simulink model "test_pi_av_formation_gazebo_final_variation"  (R2023a)
settings: Solver=FixedStepAuto  StartTime=0.0  StopTime=inf  FixedStep=0.07  RelTol=1e-3
undefined symbols (not defined in the file or in its folder): angular, DiscIntNeverNeededParam, linear
libraries: ros2lib x14, simulink x4, robotcorelib x4
(part 2 of 2)

== matlab function test_pi_av_formation_gazebo_final_variation/Translational Control2/Flocking1/MATLAB Function2 ==
  data: ui_prev input; xi input; yi input; zi input; ui_gamma output; xr input; yr input; zr input; xr2 input; yr2 input; zr2 input; fig input; iep input size=3; norm_ex input; norm_ey input; norm_ez input; ep output size=3; K_cts input

function [ui_gamma, ep] = naviFeedback(ui_prev, xi, yi, zi, xr, yr, zr, xr2, yr2, zr2, fig, iep, norm_ex, norm_ey, norm_ez, K_cts)
    
    Kpxy = K_cts(1); Kixy = K_cts(2);
    xmin_xy = K_cts(3); xmax_xy = K_cts(4);
    Kpz = K_cts(5); Kiz = K_cts(6);
    xmin_z = K_cts(7); xmax_z = K_cts(8);

    %Sepration control
    ui_xprev = ui_prev(1); ui_yprev = ui_prev(2); ui_zprev = ui_prev(3);
    
    if fig == 1
        e_x = (xr - xi - 0.5) + (xr2 - xi - 1);
        e_y = (yr - yi + 0.5) + (yr2 - yi + 1);
        e_z = (zr - zi - 0.1) + (zr2 - zi);
    elseif fig == 2
        e_x = (xr - xi - 0.5) + (xr2 - xi - 1);
        e_y = (yr - yi - 0.5) + (yr2 - yi - 1);
        e_z = (zr - zi + 0.1) + (zr2 - zi);
    else
        e_x = (xr - xi - 0.5) + (xr2 - xi - 1);
        e_y = (yr - yi - 0.5) + (yr2 - yi - 1);
        e_z = (zr - zi + 0.1) + (zr2 - zi);
    end

    e_xy = [e_x;e_y];
    ep = [e_xy;e_z];
    
    if  norm_ex >= 0
        ui_gammax = satFcn_esc(Kpxy*e_x, xmin_xy, xmax_xy) + satFcn_esc(Kixy*iep(1), xmin_xy, xmax_xy);
    else
        ui_gammax = ui_xprev;
    end

    if  norm_ey >= 0
        ui_gammay = satFcn_esc(Kpxy*e_y, xmin_xy, xmax_xy) + satFcn_esc(Kixy*iep(1), xmin_xy, xmax_xy);
    else
        ui_gammay = ui_yprev;
    end

    if  norm_ez >= 0
        ui_gammaz = satFcn_esc(Kpz*e_z, xmin_z, xmax_z) + satFcn_esc(Kiz*iep(3), xmin_z, xmax_z);
    else
        ui_gammaz = ui_zprev;
    end
    

    ui_gamma = [ui_gammax;ui_gammay;ui_gammaz];
    
end

== matlab function test_pi_av_formation_gazebo_final_variation/Translational Control3/Flocking1/MATLAB Function ==
  data: xi input; yi input; phiAlpha output; xj input; yj input; xk input; yk input; xl input; yl input; params input

function phiAlpha  = phiAlphaFcn(xi, yi, xj, yj, xk, yk, xl, yl, params)
    
    % Flocking parameters
    epsilon = params(1); a = params(2); b = params(3); c = params(4); d = params(5); h = params(6);

    e = abs(a - b) / sqrt(4*a*b) ;

    cAlpha = sigmaNormFun(c, epsilon) ;
    dAlpha = sigmaNormFun(d, epsilon) ;

    %%
    Pi = [xi;yi] ;
    Pj = [xj;yj] ;
    Pk = [xk;yk] ;
    Pl = [xl;yl] ;

    %%
    sigmaNormj = sigmaNormFun(Pj - Pi, epsilon) ;
    nij = gradSigmaFun(Pj - Pi, epsilon) ;
    
    sigmaNormk = sigmaNormFun(Pk - Pi, epsilon) ;
    nik = gradSigmaFun(Pk - Pi, epsilon) ;

    sigmaNorml = sigmaNormFun(Pl - Pi, epsilon) ;
    nil = gradSigmaFun(Pl - Pi, epsilon) ;

    %%
    sigma1j = sigma1Fun(sigmaNormj - dAlpha + e) ;
    sigma1k = sigma1Fun(sigmaNormk - dAlpha + e) ;
    sigma1l = sigma1Fun(sigmaNorml - dAlpha + e) ;
            
    %% Position
    phiAlphaj = 0.5 * bumpFcn(sigmaNormj/cAlpha,h) * ((a+b)*sigma1j + (a-b)) ;
    phiAlphanij = phiAlphaj.* nij ;
    
    phiAlphak = 0.5 * bumpFcn(sigmaNormk/cAlpha,h) * ((a+b)*sigma1k + (a-b)) ;
    phiAlphanik = phiAlphak.* nik ;

    phiAlphal = 0.5 * bumpFcn(sigmaNorml/cAlpha,h) * ((a+b)*sigma1l + (a-b)) ;
    phiAlphanil = phiAlphal.* nil ;

    phiAlpha = phiAlphanij + phiAlphanik + phiAlphanil;

    
end

== matlab function test_pi_av_formation_gazebo_final_variation/Translational Control3/Flocking1/MATLAB Function1 ==
  data: eta input; phiAlpha input; phiAlpha_int input; ui_gamma input; yaw input; Ui_pos output size=3; ui_yaw output; KP input; eyaw output size=1; eyaw1 input; eyaw2 input; eyaw4 input

function [Ui_pos, ui_yaw, eyaw]  = ctrlLaw(eta, phiAlpha, phiAlpha_int, ui_gamma, yaw, KP, eyaw1, eyaw2, eyaw4)  %, phiBetak, bikobs, phiBetanei, bikve
    
    % Control gains and parameters
    Kx = KP(1); Ky = KP(2); Kz = KP(3);
    Kix = KP(4); Kiy = KP(5); Kiz = KP(6);
    Kyaw = KP(7); Kdyaw = KP(8);
    off = KP(9);

    eyaw = 0 - yaw(1);
    deyaw = 0 - yaw(2);


    ui_yaw = Kyaw*eyaw + Kdyaw*deyaw;
    hz_dot = ui_gamma(3,1) - eta(3,1);  %+ cBetaz * (phiBetak(3,1) + phiBetanei(3,1)) + cdBetaz * (bikobs(3,1) + bikve(3,1));

    if eyaw < off && eyaw > -off % && eyaw1 < off && eyaw1 > -off && eyaw2 < off && eyaw2 > -off && eyaw4 < off && eyaw4 > -off
        hx_dot = Kx * phiAlpha(1,1) + Kix * phiAlpha_int(1,1) + ui_gamma(1,1) - eta(1,1);  %+ cBetax * (phiBetak(1,1) + phiBetanei(1,1)) + cdBetax * (bikobs(1,1) + bikve(1,1));
        hy_dot = Ky * phiAlpha(2,1) + Kiy * phiAlpha_int(2,1) + ui_gamma(2,1) - eta(2,1);  %+ cBetay * (phiBetak(2,1) + phiBetanei(2,1)) + cdBetay * (bikobs(2,1) + bikve(2,1));
    else
        hx_dot = 0;
        hy_dot = 0;
    end
    

    Ui_pos = [hx_dot; hy_dot; hz_dot] ;
    

end

== matlab function test_pi_av_formation_gazebo_final_variation/Translational Control3/Flocking1/MATLAB Function2 ==
  data: ui_prev input; xi input; yi input; zi input; ui_gamma output; xr input; yr input; zr input; xr2 input; yr2 input; zr2 input; fig input; iep input size=3; norm_ex input; norm_ey input; norm_ez input; ep output size=3; K_cts input
function [ui_gamma, ep] = naviFeedback(ui_prev, xi, yi, zi, xr, yr, zr, xr2, yr2, zr2, fig, iep, norm_ex, norm_ey, norm_ez, K_cts)
    
    Kpxy = K_cts(1); Kixy = K_cts(2);
    xmin_xy = K_cts(3); xmax_xy = K_cts(4);
    Kpz = K_cts(5); Kiz = K_cts(6);
    xmin_z = K_cts(7); xmax_z = K_cts(8);

    %Sepration control
    ui_xprev = ui_prev(1); ui_yprev = ui_prev(2); ui_zprev = ui_prev(3);

    
    if fig == 1
        e_x = (xr - xi - 0.5) + (xr2 - xi - 1);
        e_y = (yr - yi - 0.5) + (yr2 - yi);
        e_z = (zr - zi + 0.1) + (zr2 - zi);
    elseif fig == 2
        e_x = (xr - xi + 0.5) + (xr2 - xi);
        e_y = (yr - yi - 0.5) + (yr2 - yi - 1);
        e_z = (zr - zi - 0.1) + (zr2 - zi);
    else
        e_x = (xr - xi + 0.5) + (xr2 - xi);
        e_y = (yr - yi - 0.5) + (yr2 - yi - 1);
        e_z = (zr - zi - 0.5) + (zr2 - zi - 0.6);
    end

    e_xy = [e_x;e_y];
    ep = [e_xy;e_z];
    
    if  norm_ex >= 0
        ui_gammax = satFcn_esc(Kpxy*e_x, xmin_xy, xmax_xy) + satFcn_esc(Kixy*iep(1), xmin_xy, xmax_xy);
    else
        ui_gammax = ui_xprev;
    end

    if  norm_ey >= 0
        ui_gammay = satFcn_esc(Kpxy*e_y, xmin_xy, xmax_xy) + satFcn_esc(Kixy*iep(1), xmin_xy, xmax_xy);
    else
        ui_gammay = ui_yprev;
    end

    if  norm_ez >= 0
        ui_gammaz = satFcn_esc(Kpz*e_z, xmin_z, xmax_z) + satFcn_esc(Kiz*iep(3), xmin_z, xmax_z);
    else
        ui_gammaz = ui_zprev;
    end
    

    ui_gamma = [ui_gammax;ui_gammay;ui_gammaz];
end

== matlab function test_pi_av_formation_gazebo_final_variation/Translational Control4/Flocking1/MATLAB Function ==
  data: xi input; yi input; phiAlpha output; xj input; yj input; xk input; yk input; xl input; yl input; params input

function phiAlpha  = phiAlphaFcn(xi, yi, xj, yj, xk, yk, xl, yl, params)
    
    % Flocking parameters
    epsilon = params(1); a = params(2); b = params(3); c = params(4); d = params(5); h = params(6);

    e = abs(a - b) / sqrt(4*a*b) ;

    cAlpha = sigmaNormFun(c, epsilon) ;
    dAlpha = sigmaNormFun(d, epsilon) ;

    %%
    Pi = [xi;yi] ;
    Pj = [xj;yj] ;
    Pk = [xk;yk] ;
    Pl = [xl;yl] ;

    %%
    sigmaNormj = sigmaNormFun(Pj - Pi, epsilon) ;
    nij = gradSigmaFun(Pj - Pi, epsilon) ;
    
    sigmaNormk = sigmaNormFun(Pk - Pi, epsilon) ;
    nik = gradSigmaFun(Pk - Pi, epsilon) ;

    sigmaNorml = sigmaNormFun(Pl - Pi, epsilon) ;
    nil = gradSigmaFun(Pl - Pi, epsilon) ;

    %%
    sigma1j = sigma1Fun(sigmaNormj - dAlpha + e) ;
    sigma1k = sigma1Fun(sigmaNormk - dAlpha + e) ;
    sigma1l = sigma1Fun(sigmaNorml - dAlpha + e) ;
            
    %% Position
    phiAlphaj = 0.5 * bumpFcn(sigmaNormj/cAlpha,h) * ((a+b)*sigma1j + (a-b)) ;
    phiAlphanij = phiAlphaj.* nij ;
    
    phiAlphak = 0.5 * bumpFcn(sigmaNormk/cAlpha,h) * ((a+b)*sigma1k + (a-b)) ;
    phiAlphanik = phiAlphak.* nik ;

    phiAlphal = 0.5 * bumpFcn(sigmaNorml/cAlpha,h) * ((a+b)*sigma1l + (a-b)) ;
    phiAlphanil = phiAlphal.* nil ;

    phiAlpha = phiAlphanij + phiAlphanik + phiAlphanil;

    
end

== matlab function test_pi_av_formation_gazebo_final_variation/Translational Control4/Flocking1/MATLAB Function1 ==
  data: eta input; phiAlpha input; phiAlpha_int input; ui_gamma input; yaw input; Ui_pos output size=3; ui_yaw output; KP input; eyaw output size=1; eyaw1 input; eyaw2 input; eyaw3 input

function [Ui_pos, ui_yaw, eyaw]  = ctrlLaw(eta, phiAlpha, phiAlpha_int, ui_gamma, yaw, KP, eyaw1, eyaw2, eyaw3)  %, phiBetak, bikobs, phiBetanei, bikve
    
    % Control gains and parameters
    Kx = KP(1); Ky = KP(2); Kz = KP(3);
    Kix = KP(4); Kiy = KP(5); Kiz = KP(6);
    Kyaw = KP(7); Kdyaw = KP(8);
    off = KP(9);

    eyaw = 0 - yaw(1);
    deyaw = 0 - yaw(2);


    ui_yaw = Kyaw*eyaw + Kdyaw*deyaw;
    hz_dot = ui_gamma(3,1) - eta(3,1);  %+ cBetaz * (phiBetak(3,1) + phiBetanei(3,1)) + cdBetaz * (bikobs(3,1) + bikve(3,1));

    if eyaw < off && eyaw > -off % && eyaw1 < off && eyaw1 > -off && eyaw2 < off && eyaw2 > -off && eyaw3 < off && eyaw3 > -off
        hx_dot = Kx * phiAlpha(1,1) + Kix * phiAlpha_int(1,1) + ui_gamma(1,1) - eta(1,1);  %+ cBetax * (phiBetak(1,1) + phiBetanei(1,1)) + cdBetax * (bikobs(1,1) + bikve(1,1));
        hy_dot = Ky * phiAlpha(2,1) + Kiy * phiAlpha_int(2,1) + ui_gamma(2,1) - eta(2,1);  %+ cBetay * (phiBetak(2,1) + phiBetanei(2,1)) + cdBetay * (bikobs(2,1) + bikve(2,1));
    else
        hx_dot = 0;
        hy_dot = 0;
    end
    

    Ui_pos = [hx_dot; hy_dot; hz_dot] ;
    

end

== matlab function test_pi_av_formation_gazebo_final_variation/Translational Control1/Flocking1/MATLAB Function ==
  data: xi input; yi input; phiAlpha output; xj input; yj input; xk input; yk input; xl input; yl input; params input

function phiAlpha  = phiAlphaFcn(xi, yi, xj, yj, xk, yk, xl, yl, params)
    
    % Flocking parameters
    epsilon = params(1); a = params(2); b = params(3); c = params(4); d = params(5); h = params(6);

    e = abs(a - b) / sqrt(4*a*b) ;

    cAlpha = sigmaNormFun(c, epsilon) ;
    dAlpha = sigmaNormFun(d, epsilon) ;

    %%
    Pi = [xi;yi] ;
    Pj = [xj;yj] ;
    Pk = [xk;yk] ;
    Pl = [xl;yl] ;

    %%
    sigmaNormj = sigmaNormFun(Pj - Pi, epsilon) ;
    nij = gradSigmaFun(Pj - Pi, epsilon) ;
    
    sigmaNormk = sigmaNormFun(Pk - Pi, epsilon) ;
    nik = gradSigmaFun(Pk - Pi, epsilon) ;

    sigmaNorml = sigmaNormFun(Pl - Pi, epsilon) ;
    nil = gradSigmaFun(Pl - Pi, epsilon) ;

    %%
    sigma1j = sigma1Fun(sigmaNormj - dAlpha + e) ;
    sigma1k = sigma1Fun(sigmaNormk - dAlpha + e) ;
    sigma1l = sigma1Fun(sigmaNorml - dAlpha + e) ;
            
    %% Position
    phiAlphaj = 0.5 * bumpFcn(sigmaNormj/cAlpha,h) * ((a+b)*sigma1j + (a-b)) ;
    phiAlphanij = phiAlphaj.* nij ;
    
    phiAlphak = 0.5 * bumpFcn(sigmaNormk/cAlpha,h) * ((a+b)*sigma1k + (a-b)) ;
    phiAlphanik = phiAlphak.* nik ;

    phiAlphal = 0.5 * bumpFcn(sigmaNorml/cAlpha,h) * ((a+b)*sigma1l + (a-b)) ;
    phiAlphanil = phiAlphal.* nil ;

    phiAlpha = phiAlphanij + phiAlphanik + phiAlphanil;

    
end

== matlab function test_pi_av_formation_gazebo_final_variation/Translational Control1/Flocking1/MATLAB Function1 ==
  data: eta input; phiAlpha input; phiAlpha_int input; ui_gamma input; yaw input; Ui_pos output size=3; ui_yaw output; KP input; eyaw output size=1; eyaw2 input; eyaw3 input; eyaw4 input

function [Ui_pos, ui_yaw, eyaw]  = ctrlLaw(eta, phiAlpha, phiAlpha_int, ui_gamma, yaw, KP, eyaw2, eyaw3, eyaw4)  %, phiBetak, bikobs, phiBetanei, bikve
    
    % Control gains and parameters
    Kx = KP(1); Ky = KP(2); Kz = KP(3);
    Kix = KP(4); Kiy = KP(5); Kiz = KP(6);
    Kyaw = KP(7); Kdyaw = KP(8);
    off = KP(9);


    eyaw = 0 - yaw(1);
    deyaw = 0 - yaw(2);


    ui_yaw = Kyaw*eyaw + Kdyaw*deyaw;
    hz_dot = ui_gamma(3,1) - eta(3,1);  %+ cBetaz * (phiBetak(3,1) + phiBetanei(3,1)) + cdBetaz * (bikobs(3,1) + bikve(3,1));

    if eyaw < off && eyaw > -off % && eyaw2 < off && eyaw2 > -off  && eyaw3 < off && eyaw3 > -off && eyaw4 < off && eyaw4 > -off
        hx_dot = Kx * phiAlpha(1,1) + Kix * phiAlpha_int(1,1) + ui_gamma(1,1) - eta(1,1);  %+ cBetax * (phiBetak(1,1) + phiBetanei(1,1)) + cdBetax * (bikobs(1,1) + bikve(1,1));
        hy_dot = Ky * phiAlpha(2,1) + Kiy * phiAlpha_int(2,1) + ui_gamma(2,1) - eta(2,1);  %+ cBetay * (phiBetak(2,1) + phiBetanei(2,1)) + cdBetay * (bikobs(2,1) + bikve(2,1));
    else
        hx_dot = 0;
        hy_dot = 0;
    end
    

    Ui_pos = [hx_dot; hy_dot; hz_dot] ;
    

end

== matlab function test_pi_av_formation_gazebo_final_variation/Translational Control1/Flocking1/MATLAB Function2 ==
  data: ui_prev input; xi input; yi input; zi input; ui_gamma output; xr input; yr input; zr input; figure input; iep input size=3; norm_ex input; norm_ey input; norm_ez input; ep output size=3; K_cts input

function [ui_gamma, ep] = naviFeedback(ui_prev, xi, yi, zi, xr, yr, zr, figure, iep, norm_ex, norm_ey, norm_ez, K_cts)
    
    Kpxy = K_cts(1); Kixy = K_cts(2);
    xmin_xy = K_cts(3); xmax_xy = K_cts(4);
    Kpz = K_cts(5); Kiz = K_cts(6);
    xmin_z = K_cts(7); xmax_z = K_cts(8);

    %Sepration control
    ui_xprev = ui_prev(1); ui_yprev = ui_prev(2); ui_zprev = ui_prev(3);

    if figure == 1
        e_x = xr - xi + 0.5;
        e_y = yr - yi + 0.5;
        e_z = zr - zi + 0.1;
    elseif figure == 2
        e_x = xr - xi - 0.5;
        e_y = yr - yi + 0.5;
        e_z = zr - zi - 0.1;
    else
        e_x = xr - xi - 0.5;
        e_y = yr - yi + 0.5;
        e_z = zr - zi - 0.5;
    end

    e_xy = [e_x;e_y];
    ep = [e_xy;e_z];
    
    if  norm_ex >= 0
        ui_gammax = satFcn_esc(Kpxy*e_x, xmin_xy, xmax_xy) + satFcn_esc(Kixy*iep(1), xmin_xy, xmax_xy);
    else
        ui_gammax = ui_xprev;
    end

    if  norm_ey >= 0
        ui_gammay = satFcn_esc(Kpxy*e_y, xmin_xy, xmax_xy) + satFcn_esc(Kixy*iep(1), xmin_xy, xmax_xy);
    else
        ui_gammay = ui_yprev;
    end

    if  norm_ez >= 0
        ui_gammaz = satFcn_esc(Kpz*e_z, xmin_z, xmax_z) + satFcn_esc(Kiz*iep(3), xmin_z, xmax_z);
    else
        ui_gammaz = ui_zprev;
    end
    

    ui_gamma = [ui_gammax;ui_gammay;ui_gammaz];
    
end

== matlab function test_pi_av_formation_gazebo_final_variation/Translational Control4/Flocking1/MATLAB Function2 ==
  data: ui_prev input; xi input; yi input; zi input; ui_gamma output; xr input; yr input; zr input; xr2 input; yr2 input; zr2 input; fig input; iep input size=3; norm_ex input; norm_ey input; norm_ez input; ep output size=3; K_cts input
function [ui_gamma, ep] = naviFeedback(ui_prev, xi, yi, zi, xr, yr, zr, xr2, yr2, zr2, fig, iep, norm_ex, norm_ey, norm_ez, K_cts)
    
    Kpxy = K_cts(1); Kixy = K_cts(2);
    xmin_xy = K_cts(3); xmax_xy = K_cts(4);
    Kpz = K_cts(5); Kiz = K_cts(6);
    xmin_z = K_cts(7); xmax_z = K_cts(8);

    %Sepration control
    ui_xprev = ui_prev(1); ui_yprev = ui_prev(2); ui_zprev = ui_prev(3);
    
    if fig == 1
        e_x = (xr - xi + 0.5) + (xr2 - xi);
        e_y = (yr - yi - 0.5) + (yr2 - yi - 1);
        e_z = (zr - zi - 0.1) + (zr2 - zi);
    elseif fig == 2
        e_x = (xr - xi + 0.5) + (xr2 - xi + 1);
        e_y = (yr - yi + 0.5) + (yr2 - yi);
        e_z = (zr - zi + 0.1) + (zr2 - zi);
    else
        e_x = (xr - xi + 0.5) + (xr2 - xi + 1);
        e_y = (yr - yi + 0.5) + (yr2 - yi);
        e_z = (zr - zi + 0.1) + (zr2 - zi);
    end

    e_xy = [e_x;e_y];
    ep = [e_xy;e_z];
    
    if  norm_ex >= 0
        ui_gammax = satFcn_esc(Kpxy*e_x, xmin_xy, xmax_xy) + satFcn_esc(Kixy*iep(1), xmin_xy, xmax_xy);
    else
        ui_gammax = ui_xprev;
    end

    if  norm_ey >= 0
        ui_gammay = satFcn_esc(Kpxy*e_y, xmin_xy, xmax_xy) + satFcn_esc(Kixy*iep(1), xmin_xy, xmax_xy);
    else
        ui_gammay = ui_yprev;
    end

    if  norm_ez >= 0
        ui_gammaz = satFcn_esc(Kpz*e_z, xmin_z, xmax_z) + satFcn_esc(Kiz*iep(3), xmin_z, xmax_z);
    else
        ui_gammaz = ui_zprev;
    end
    

    ui_gamma = [ui_gammax;ui_gammay;ui_gammaz];
end

== matlab function test_pi_av_formation_gazebo_final_variation/Translational Control1/Flocking1/MATLAB Function5 ==
  data: dot_hat_q output; L input; q input; q_hat input; eta1 input; u input; dot_eta output
function [dot_hat_q, dot_eta] = fcn(L, q, q_hat, eta1, u)

%%separation gains vectors
l1 = [L(1) L(2) L(3)];
l0 = [L(4) L(5) L(6)];

L_1 = diag(l1);
L_0 = diag(l0);

dot_hat_q = q_est(u, eta1, L_1, q, q_hat);

dot_eta = dot_eta_two(L_0, q, q_hat);

== matlab function test_pi_av_formation_gazebo_final_variation/Translational Control2/Flocking1/MATLAB Function5 ==
  data: dot_hat_q output; L input; q input; q_hat input; eta1 input; u input; dot_eta output
function [dot_hat_q, dot_eta] = fcn(L, q, q_hat, eta1, u)

%%separation gains vectors
l1 = [L(1) L(2) L(3)];
l0 = [L(4) L(5) L(6)];

L_1 = diag(l1);
L_0 = diag(l0);

dot_hat_q = q_est(u, eta1, L_1, q, q_hat);

dot_eta = dot_eta_two(L_0, q, q_hat);

== matlab function test_pi_av_formation_gazebo_final_variation/Translational Control3/Flocking1/MATLAB Function5 ==
  data: dot_hat_q output; L input; q input; q_hat input; eta1 input; u input; dot_eta output
function [dot_hat_q, dot_eta] = fcn(L, q, q_hat, eta1, u)

%%separation gains vectors
l1 = [L(1) L(2) L(3)];
l0 = [L(4) L(5) L(6)];

L_1 = diag(l1);
L_0 = diag(l0);

dot_hat_q = q_est(u, eta1, L_1, q, q_hat);

dot_eta = dot_eta_two(L_0, q, q_hat);

== matlab function test_pi_av_formation_gazebo_final_variation/Translational Control4/Flocking1/MATLAB Function5 ==
  data: dot_hat_q output; L input; q input; q_hat input; eta1 input; u input; dot_eta output
function [dot_hat_q, dot_eta] = fcn(L, q, q_hat, eta1, u)

%%separation gains vectors
l1 = [L(1) L(2) L(3)];
l0 = [L(4) L(5) L(6)];

L_1 = diag(l1);
L_0 = diag(l0);

dot_hat_q = q_est(u, eta1, L_1, q, q_hat);

dot_eta = dot_eta_two(L_0, q, q_hat);

== matlab function test_pi_av_formation_gazebo_final_variation/Translational Control1/Flocking1/event_x2 ==
  data: e_1 output; e_2 output; e1 input; e2 input; e3 input; e_3 output; i1 output; i1 input; i2 input; i3 input; i2 output; i3 output
function [e_1,e_2, e_3, i1, i2, i3]  = fcn(e1, e2, e3, i1, i2, i3)

if e1 >= 0
    e_1 = 1;
    i1 = i1+1;
else 
    e_1 = 0;
    i1 = i1;
end

if e2 >= 0
    e_2 = 1;
    i2 = i2 + 1;
else 
    e_2 = 0;
    i2 = i2;
end

if e3 >= 0
    e_3 = 1;
    i3 = i3 + 1;
else 
    e_3 = 0;
    i3 = i3;
end

== matlab function test_pi_av_formation_gazebo_final_variation/Translational Control1/Flocking1/event_1 ==
  data: x input; y input; z input; mx input; my input; mz input; norm_ex output; norm_ey output; c0 input; norm_ez output
function [norm_ex, norm_ey, norm_ez] = fcn(x, y, z, mx, my, mz, c0)

cx = c0(1); cy = c0(2); cz = c0(3); 

norm_ex = abs((mx-x)) - cx;
norm_ey = abs((my-y)) - cy;
norm_ez = abs((mz-z)) - cz;

== matlab function test_pi_av_formation_gazebo_final_variation/Translational Control1/Flocking1/memory_1 ==
  data: ex input; ey input; mx output; ez input; x input; y input; z input; mx input; my input; mz input; my output; mz output
function [mx, my, mz] = fcn(ex, ey, ez, x, y, z, mx, my, mz)

if ex >= 0
    mx = x;    
else
    mx = mx;
end

if ey >= 0
    my = y;    
else
    my = my;
end

if ez >= 0
    mz = z;    
else
    mz = mz;
end

== matlab function test_pi_av_formation_gazebo_final_variation/Translational Control2/Flocking1/event_1 ==
  data: x input; y input; z input; mx input; my input; mz input; norm_ex output; norm_ey output; c0 input; norm_ez output
function [norm_ex, norm_ey, norm_ez] = fcn(x, y, z, mx, my, mz, c0)

cx = c0(1); cy = c0(2); cz = c0(3); 

norm_ex = abs((mx-x)) - cx;
norm_ey = abs((my-y)) - cy;
norm_ez = abs((mz-z)) - cz;

== matlab function test_pi_av_formation_gazebo_final_variation/Translational Control2/Flocking1/memory_1 ==
  data: ex input; ey input; mx output; ez input; x input; y input; z input; mx input; my input; mz input; my output; mz output
function [mx, my, mz] = fcn(ex, ey, ez, x, y, z, mx, my, mz)

if ex >= 0
    mx = x;    
else
    mx = mx;
end

if ey >= 0
    my = y;    
else
    my = my;
end

if ez >= 0
    mz = z;    
else
    mz = mz;
end

== matlab function test_pi_av_formation_gazebo_final_variation/Translational Control3/Flocking1/event_1 ==
  data: x input; y input; z input; mx input; my input; mz input; norm_ex output; norm_ey output; c0 input; norm_ez output
function [norm_ex, norm_ey, norm_ez] = fcn(x, y, z, mx, my, mz, c0)

cx = c0(1); cy = c0(2); cz = c0(3); 

norm_ex = abs((mx-x)) - cx;
norm_ey = abs((my-y)) - cy;
norm_ez = abs((mz-z)) - cz;

== matlab function test_pi_av_formation_gazebo_final_variation/Translational Control3/Flocking1/memory_1 ==
  data: ex input; ey input; mx output; ez input; x input; y input; z input; mx input; my input; mz input; my output; mz output
function [mx, my, mz] = fcn(ex, ey, ez, x, y, z, mx, my, mz)

if ex >= 0
    mx = x;    
else
    mx = mx;
end

if ey >= 0
    my = y;    
else
    my = my;
end

if ez >= 0
    mz = z;    
else
    mz = mz;
end

== matlab function test_pi_av_formation_gazebo_final_variation/Translational Control4/Flocking1/event_1 ==
  data: x input; y input; z input; mx input; my input; mz input; norm_ex output; norm_ey output; c0 input; norm_ez output
function [norm_ex, norm_ey, norm_ez] = fcn(x, y, z, mx, my, mz, c0)

cx = c0(1); cy = c0(2); cz = c0(3); 

norm_ex = abs((mx-x)) - cx;
norm_ey = abs((my-y)) - cy;
norm_ez = abs((mz-z)) - cz;

== matlab function test_pi_av_formation_gazebo_final_variation/Translational Control4/Flocking1/memory_1 ==
  data: ex input; ey input; mx output; ez input; x input; y input; z input; mx input; my input; mz input; my output; mz output
function [mx, my, mz] = fcn(ex, ey, ez, x, y, z, mx, my, mz)

if ex >= 0
    mx = x;    
else
    mx = mx;
end

if ey >= 0
    my = y;    
else
    my = my;
end

if ez >= 0
    mz = z;    
else
    mz = mz;
end

== matlab function test_pi_av_formation_gazebo_final_variation/Subsystem/dist_AVT ==
  data: meas input; u_B input; dU output; dAVT output; avt_pars input
function [dU,dAVT]  = fcn(meas, u_B, avt_pars)

%Vector separation
d1 = meas(1);
d2 = meas(2);
d3 = meas(3);

avtpars = avt_pars(1:4);
inc = avtpars(1);
dec = avtpars(2);
min = avtpars(3);
max = avtpars(4);

%% memory variables
d_avt1 = u_B(1);
adjustment1 = u_B(2);
s_adjust1 = u_B(3);

d_avt2 = u_B(4);
adjustment2 = u_B(5);
s_adjust2 = u_B(6);

d_avt3 = u_B(7);
adjustment3 = u_B(8);
s_adjust3 = u_B(9);

%%
du1 = AVTfun(d_avt1, d1, adjustment1, s_adjust1, min, max, inc, dec);

du2 = AVTfun(d_avt2, d2, adjustment2, s_adjust2, min, max, inc, dec);

du3 = AVTfun(d_avt3, d3, adjustment3, s_adjust3, min, max, inc, dec);

dU = [du1;du2;du3];
dAVT = [du1(1);du2(1);du3(1)];

== matlab function test_pi_av_formation_gazebo_final_variation/Subsystem/MATLAB Function6 ==
  data: X1 input; X2 input; X3 input; d_meas input; xyz output
function xyz = fcn(X1, X2, X3, d_meas)

%% Extract data from vectors
states1 = X1(1:3);
x1 = states1(1);
y1 = states1(2);
z1 = states1(3);

states2 = X2(1:3);
x2 = states2(1);
y2 = states2(2);
z2 = states2(3);

states3 = X3(1:3);
x3 = states3(1);
y3 = states3(2);
z3 = states3(3);

r1 = d_meas(1);
r2 = d_meas(2);
r3 = d_meas(3);

xyz = multi_fun(x1, y1, r1, x2, y2, r2, x3, y3, r3);

== matlab function test_pi_av_formation_gazebo_final_variation/Translational Control2/Flocking1/event_x2 ==
  data: e1 input; e2 input; e3 input; i1 output; i1 input; i2 input; i3 input; i2 output; i3 output
function [i1, i2, i3]  = fcn(e1, e2, e3, i1, i2, i3)

if e1 >= 0
    e_1 = 1;
    i1 = i1+1;
else 
    e_1 = 0;
    i1 = i1;
end

if e2 >= 0
    e_2 = 1;
    i2 = i2 + 1;
else 
    e_2 = 0;
    i2 = i2;
end

if e3 >= 0
    e_3 = 1;
    i3 = i3 + 1;
else 
    e_3 = 0;
    i3 = i3;
end

== matlab function test_pi_av_formation_gazebo_final_variation/Translational Control3/Flocking1/event_x2 ==
  data: e1 input; e2 input; e3 input; i1 output; i1 input; i2 input; i3 input; i2 output; i3 output
function [i1, i2, i3]  = fcn(e1, e2, e3, i1, i2, i3)

if e1 >= 0
    e_1 = 1;
    i1 = i1+1;
else 
    e_1 = 0;
    i1 = i1;
end

if e2 >= 0
    e_2 = 1;
    i2 = i2 + 1;
else 
    e_2 = 0;
    i2 = i2;
end

if e3 >= 0
    e_3 = 1;
    i3 = i3 + 1;
else 
    e_3 = 0;
    i3 = i3;
end

== matlab function test_pi_av_formation_gazebo_final_variation/Translational Control4/Flocking1/event_x2 ==
  data: e1 input; e2 input; e3 input; i1 output; i1 input; i2 input; i3 input; i2 output; i3 output
function [i1, i2, i3]  = fcn(e1, e2, e3, i1, i2, i3)

if e1 >= 0
    e_1 = 1;
    i1 = i1+1;
else 
    e_1 = 0;
    i1 = i1;
end

if e2 >= 0
    e_2 = 1;
    i2 = i2 + 1;
else 
    e_2 = 0;
    i2 = i2;
end

if e3 >= 0
    e_3 = 1;
    i3 = i3 + 1;
else 
    e_3 = 0;
    i3 = i3;
end

== matlab function test_pi_av_formation_gazebo_final_variation/MATLAB Function1 ==
  data: sec input; gaz_time output; nanosec input
function gaz_time = fcn(sec, nanosec)

nanosec1 = double(nanosec)/1000000000; %*10^(-9);

sec1 = double(sec);

gaz_time = sec1 + nanosec1;
